simulink model "controller_autogen"  (R2022b)
settings: Solver=FixedStepDiscrete  StartTime=0.0  StopTime=inf  FixedStep=0.005  RelTol=1e-3
undefined symbols (not defined in the file): MI_STATUSES, simp_vd_interface, simp_vd_lib
libraries: battery_monitor_lib x1, driver_interface_lib x1, governor_lib x1, motor_interface_lib x1
settings Model: Creator=dr_pa  LastModifiedBy=LinF
settings OptimizationCC: DefaultParameterBehavior=Inlined  UseDivisionForNetSlopeComputation=on  GainParamInheritBuiltInType=on  UseFloatMulNetSlope=on  InlineInvariantSignals=on  PassReuseOutputArgsAs=Individual arguments  ZeroExternalMemoryAtStartup=off  ZeroInternalMemoryAtStartup=off  NoFixptDivByZeroProtection=on  EfficientFloat2IntCast=on  LifeSpan=1  OptimizeBlockOrder=speed  DifferentSizesBufferReuse=on  EfficientTunableParamExpr=on
settings DebuggingCC: ParameterTunabilityLossMsg=error
settings HardwareCC: ProdBitPerPointer=32  ProdBitPerSizeT=32  ProdBitPerPtrDiffT=32  ProdLargestAtomicInteger=Long  ProdLargestAtomicFloat=Double  ProdWordSize=32  ProdLongLongMode=on  ProdHWDeviceType=ARM Compatible->ARM Cortex-M
settings SFSimCC: MATLABDynamicMemAlloc=off
settings RTWCC: Description=Embedded Coder  SystemTargetFile=ert.tlc  GenCodeOnly=on  TemplateMakefile=ert_default_tmf
settings CodeAppCC: ForceParamTrailComments=on  IgnoreCustomStorageClasses=off  OperatorAnnotations=on  SimulinkDataObjDesc=on  SFDataObjDesc=on  CustomSymbolStrGlobalVar=rt$N$M  CustomSymbolStrType=$N$M  CustomSymbolStrFcn=$N$M$F  CustomSymbolStrMacro=$N$M  InsertBlockDesc=on
settings ERTTargetCC: TargetLangStandard=C99 (ISO)  IncludeMdlTerminateFcn=off  CombineSignalStateStructs=on  SupportAbsoluteTime=off  SupportComplex=off  SupportNonInlinedSFcns=on  InlinedParameterPlacement=NonHierarchical  ERTCustomFileTemplate=example_file_process.tlc  ERTFilePackagingFormat=CompactWithDataFile

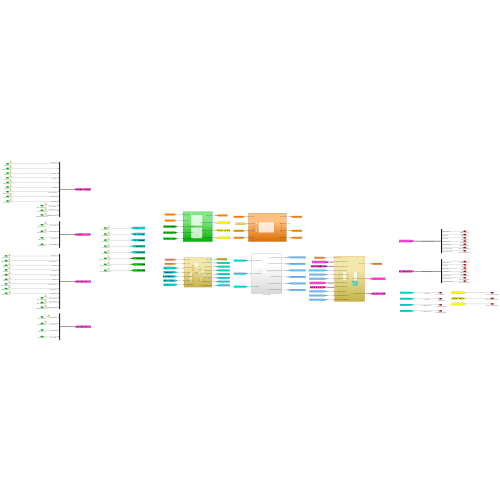
[thumbnail: Simulink's stored preview of the top-level diagram]
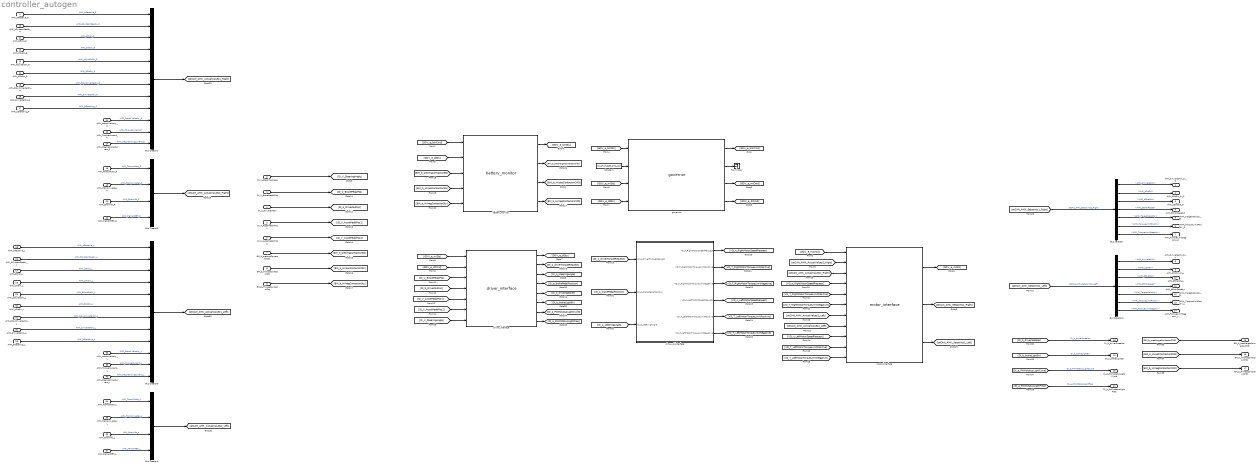
== system controller_autogen ==
  AMK_bReserve_R : Inport  OutDataTypeStr=boolean  Unit=uint64
  DI_V_SteeringAngle : Inport  Port=2  Unit=uint32
  DI_V_BrakePedalPos : Inport  Port=3  Unit=uint32
  DI_b_DriverButton : Inport  Port=4  Unit=uint32
  DI_V_AccelPedalPos1 : Inport  Port=5  Unit=uint32
  DI_V_AccelPedalPos2 : Inport  Port=6  Unit=uint32
  BM_b_prechrgContactorSts : Inport  Port=7  Unit=uint32
  BM_b_HVposContactorSts : Inport  Port=8  Unit=uint32
  BM_b_HVnegContactorSts : Inport  Port=9  Unit=uint32
  AMK_bSystemReady_R : Inport  Port=10  OutDataTypeStr=boolean  Unit=uint64
  AMK_bError_R : Inport  Port=11  OutDataTypeStr=boolean  Unit=uint64
  AMK_bWarn_R : Inport  Port=12  OutDataTypeStr=boolean  Unit=uint64
  AMK_bQuitDcOn_R : Inport  Port=13  OutDataTypeStr=boolean  Unit=uint64
  AMK_bDcOn_R : Inport  Port=14  OutDataTypeStr=boolean  Unit=uint64
  AMK_bQuitInverterOn_R : Inport  Port=15  OutDataTypeStr=boolean  Unit=uint64
  AMK_bInverterOn_R : Inport  Port=16  OutDataTypeStr=boolean  Unit=uint64
  AMK_bDerating_R : Inport  Port=17  OutDataTypeStr=boolean  Unit=uint64
  AMK_TempMotor_R : Inport  Port=18  OutDataTypeStr=int16  Unit=uint64
  AMK_TempInverter_R : Inport  Port=19  OutDataTypeStr=int16  Unit=uint64
  AMK_ErrorInfo_R : Inport  Port=20  OutDataTypeStr=uint16
  AMK_TempIGBT_R : Inport  Port=21  OutDataTypeStr=int16
  AMK_ActualVelocity_R : Inport  Port=22  OutDataTypeStr=int16  Unit=uint64
  AMK_TorqueCurrent_R : Inport  Port=23  OutDataTypeStr=int16  Unit=uint64
  AMK_MagnetizingCurrent_R : Inport  Port=24  OutDataTypeStr=int16  Unit=uint64
  AMK_bReserve_L : Inport  Port=25  OutDataTypeStr=boolean  Unit=uint64
  AMK_bSystemReady_L : Inport  Port=26  OutDataTypeStr=boolean  Unit=uint64
  AMK_bError_L : Inport  Port=27  OutDataTypeStr=boolean  Unit=uint64
  AMK_bWarn_L : Inport  Port=28  OutDataTypeStr=boolean  Unit=uint64
  AMK_bQuitDcOn_L : Inport  Port=29  OutDataTypeStr=boolean  Unit=uint64
  AMK_bDcOn_L : Inport  Port=30  OutDataTypeStr=boolean  Unit=uint64
  AMK_bQuitInverterOn_L : Inport  Port=31  OutDataTypeStr=boolean  Unit=uint64
  AMK_bInverterOn_L : Inport  Port=32  OutDataTypeStr=boolean  Unit=uint64
  AMK_bDerating_L : Inport  Port=33  OutDataTypeStr=boolean  Unit=uint64
  AMK_TempMotor_L : Inport  Port=34  OutDataTypeStr=int16  Unit=uint64
  AMK_TempInverter_L : Inport  Port=35  OutDataTypeStr=int16  Unit=uint64
  AMK_ErrorInfo_L : Inport  Port=36  OutDataTypeStr=uint16
  AMK_TempIGBT_L : Inport  Port=37  OutDataTypeStr=int16
  AMK_ActualVelocity_L : Inport  Port=38  OutDataTypeStr=int16  Unit=uint64
  AMK_TorqueCurrent_L : Inport  Port=39  OutDataTypeStr=int16  Unit=uint64
  AMK_MagnetizingCurrent_L : Inport  Port=40  OutDataTypeStr=int16  Unit=uint64
  Bus Creator1 : BusCreator  Inputs=12
  Bus Creator2 : BusCreator  Inputs=4
  Bus Creator3 : BusCreator  Inputs=12
  Bus Creator4 : BusCreator  Inputs=4
  Bus Selector : BusSelector  OutputSignals=AMK_bInverterOn,AMK_bDcOn,AMK_bEnable,AMK_bErrorReset,AMK_TargetVelocity,AMK_TorqueLimitPositiv,AMK_TorqueLimitNegativ
  Bus Selector1 : BusSelector  OutputSignals=AMK_bInverterOn,AMK_bDcOn,AMK_bEnable,AMK_bErrorReset,AMK_TargetVelocity,AMK_TorqueLimitPositiv,AMK_TorqueLimitNegativ
  Constant : Constant  Value=MI_STATUSES.STS_INIT  OutDataTypeStr=Enum: MI_STATUSES
  Terminator : Terminator
  battery_monitor : battery_monitor_lib/battery_monitor  SystemSampleTime=-1  VariantActivationTime=update diagram  Latency=0  AutoFrameSizeCalculation=off
  driver_interface : driver_interface_lib/driver_interface  SystemSampleTime=-1  VariantActivationTime=update diagram  Latency=0  AutoFrameSizeCalculation=off
  governor : governor_lib/governor  SystemSampleTime=-1  VariantActivationTime=update diagram  Latency=0  AutoFrameSizeCalculation=off
  motor_interface : motor_interface_lib/motor_interface  SystemSampleTime=-1  VariantActivationTime=update diagram  Latency=0  AutoFrameSizeCalculation=off
  simp_vd_interface : Subsystem  AncestorBlock=simp_vd_lib/simp_vd_interface
      settings: LibrarySourceBlock=simp_vd_lib/simp_vd_interface
  AMK_bInverterOn_tx_R : Outport
  AMK_bDcOn_tx_R : Outport  Port=2
  AMK_bEnable_R : Outport  Port=3
  AMK_bErrorReset_R : Outport  Port=4
  AMK_TargetVelocity_R : Outport  Port=5
  AMK_TorqueLimitPositiv_R : Outport  Port=6
  AMK_TorqueLimitNegativ_R : Outport  Port=7
  AMK_bInverterOn_tx_L : Outport  Port=8
  AMK_bDcOn_tx_L : Outport  Port=9
  AMK_bEnable_L : Outport  Port=10
  AMK_bErrorReset_L : Outport  Port=11
  AMK_TargetVelocity_L : Outport  Port=12
  AMK_TorqueLimitPositiv_L : Outport  Port=13
  AMK_TorqueLimitNegativ_L : Outport  Port=14
  BM_b_prechargeContactorCMD : Outport  Port=15
  BM_b_HVposContactorCMD : Outport  Port=16
  BM_b_HVnegContactorCMD : Outport  Port=17
  DI_b_driverSpeaker : Outport  Port=18
  DI_b_brakeLightEn : Outport  Port=19
  DI_p_PWMstatusLightCycle : Outport  Port=20
  DI_p_PWMstatusLightFreq : Outport  Port=21
  wires:
  driver_interface/3 -> [DI_p_steeringAngle]
  driver_interface/5 -> [DI_b_driverSpeaker]
  [GOV_e_miSts] -> governor/3
  [VD_T_RightMotorTorqueLimitPositive] -> motor_interface/5
  driver_interface/4 -> [DI_p_brakePedalPosition]
  BM_b_HVnegContactorSts/1 -> [BM_b_HVnegContactorSts]
  [ptCAN_AMK_Setpoints1_Left] -> Bus Selector1/1  "ptCAN_AMK_Setpoints1_Left"
  [DI_b_driverSpeaker] -> DI_b_driverSpeaker/1  "DI_b_driverSpeaker"
  [VD_T_RightMotorTorqueLimitNegative] -> motor_interface/6
  [GOV_e_bmCmd] -> battery_monitor/1
  driver_interface/2 -> [DI_p_driverTorqueRequest]
  DI_V_BrakePedalPos/1 -> [DI_V_BrakePedalPos]
  driver_interface/1 -> [GOV_e_diSts]
  Constant/1 -> governor/2
  [ptCAN_AMK_ActualValues2_Right] -> motor_interface/3
  [GOV_e_bmSts] -> governor/1
  battery_monitor/1 -> [GOV_e_bmSts]
  [VD_n_RightMotorSpeedRequest] -> motor_interface/4
  DI_V_AccelPedalPos2/1 -> [DI_V_AccelPedalPos2]
  governor/3 -> [GOV_e_miCmd]
  [GOV_e_diSts] -> governor/4
  [ptCAN_AMK_Setpoints1_Right] -> Bus Selector/1  "ptCAN_AMK_Setpoints1_Right"
  DI_b_DriverButton/1 -> [DI_b_DriverButton]
  BM_b_prechrgContactorSts/1 -> [BM_b_prechrgContactorSts]
  [GOV_e_miCmd] -> motor_interface/1
  governor/4 -> [GOV_e_diCmd]
  [ptCAN_AMK_ActualValues1_Right] -> motor_interface/2
  DI_V_AccelPedalPos1/1 -> [DI_V_AccelPedalPos1]
  governor/2 -> Terminator/1
  motor_interface/1 -> [GOV_e_miSts]
  BM_b_HVposContactorSts/1 -> [BM_b_HVposContactorSts]
  governor/1 -> [GOV_e_bmCmd]
  motor_interface/2 -> [ptCAN_AMK_Setpoints1_Right]
  DI_V_SteeringAngle/1 -> [DI_V_SteeringAngle]
  AMK_bSystemReady_R/1 -> Bus Creator1/2  "AMK_bSystemReady_R"
  AMK_bDerating_R/1 -> Bus Creator1/9  "AMK_bDerating_R"
  Bus Creator1/1 -> [ptCAN_AMK_ActualValues1_Right]
  AMK_bQuitDcOn_R/1 -> Bus Creator1/5  "AMK_bQuitDcOn_R"
  AMK_bQuitInverterOn_R/1 -> Bus Creator1/7  "AMK_bQuitInverterOn_R"
  AMK_TempInverter_R/1 -> Bus Creator2/2  "AMK_TempInverter_R"
  AMK_bDcOn_R/1 -> Bus Creator1/6  "AMK_bDcOn_R"
  AMK_bReserve_R/1 -> Bus Creator1/1  "AMK_bReserve_R"
  AMK_bWarn_R/1 -> Bus Creator1/4  "AMK_bWarn_R"
  AMK_ActualVelocity_R/1 -> Bus Creator1/10  "AMK_ActualVelocity_R"
  AMK_bError_R/1 -> Bus Creator1/3  "AMK_bError_R"
  AMK_TempMotor_R/1 -> Bus Creator2/1  "AMK_TempMotor_R"
  AMK_TorqueCurrent_R/1 -> Bus Creator1/11  "AMK_TorqueCurrent_R"
  AMK_TempIGBT_R/1 -> Bus Creator2/4  "AMK_TempIGBT_R"
  AMK_ErrorInfo_R/1 -> Bus Creator2/3  "AMK_ErrorInfo_R"
  AMK_MagnetizingCurrent_R/1 -> Bus Creator1/12  "AMK_MagnetizingCurrent_R"
  Bus Creator2/1 -> [ptCAN_AMK_ActualValues2_Right]
  AMK_bInverterOn_R/1 -> Bus Creator1/8  "AMK_bInverterOn_R"
  motor_interface/3 -> [ptCAN_AMK_Setpoints1_Left]
  [ptCAN_AMK_ActualValues1_Left] -> motor_interface/7
  [ptCAN_AMK_ActualValues2_Left] -> motor_interface/8
  [VD_n_LeftMotorSpeedRequest] -> motor_interface/9
  [VD_T_LeftMotorTorqueLimitPositive] -> motor_interface/10
  [VD_T_LeftMotorTorqueLimitNegative] -> motor_interface/11
  Bus Selector/4 -> AMK_bErrorReset_R/1  "<AMK_bErrorReset>"
  Bus Selector/5 -> AMK_TargetVelocity_R/1  "<AMK_TargetVelocity>"
  Bus Selector/1 -> AMK_bInverterOn_tx_R/1  "<AMK_bInverterOn>"
  Bus Selector/2 -> AMK_bDcOn_tx_R/1  "<AMK_bDcOn>"
  Bus Selector/6 -> AMK_TorqueLimitPositiv_R/1  "<AMK_TorqueLimitPositiv>"
  Bus Selector/3 -> AMK_bEnable_R/1  "<AMK_bEnable>"
  Bus Selector/7 -> AMK_TorqueLimitNegativ_R/1  "<AMK_TorqueLimitNegativ>"
  AMK_TorqueCurrent_L/1 -> Bus Creator3/11  "AMK_TorqueCurrent_L"
  AMK_ErrorInfo_L/1 -> Bus Creator4/3  "AMK_ErrorInfo_L"
  Bus Creator4/1 -> [ptCAN_AMK_ActualValues2_Left]
  AMK_bQuitInverterOn_L/1 -> Bus Creator3/7  "AMK_bQuitInverterOn_L"
  AMK_bSystemReady_L/1 -> Bus Creator3/2  "AMK_bSystemReady_L"
  AMK_MagnetizingCurrent_L/1 -> Bus Creator3/12  "AMK_MagnetizingCurrent_L"
  AMK_TempInverter_L/1 -> Bus Creator4/2  "AMK_TempInverter_L"
  AMK_bDerating_L/1 -> Bus Creator3/9  "AMK_bDerating_L"
  AMK_bQuitDcOn_L/1 -> Bus Creator3/5  "AMK_bQuitDcOn_L"
  AMK_TempIGBT_L/1 -> Bus Creator4/4  "AMK_TempIGBT_L"
  AMK_bDcOn_L/1 -> Bus Creator3/6  "AMK_bDcOn_L"
  AMK_TempMotor_L/1 -> Bus Creator4/1  "AMK_TempMotor_L"
  Bus Creator3/1 -> [ptCAN_AMK_ActualValues1_Left]
  AMK_bError_L/1 -> Bus Creator3/3  "AMK_bError_L"
  AMK_bWarn_L/1 -> Bus Creator3/4  "AMK_bWarn_L"
  AMK_ActualVelocity_L/1 -> Bus Creator3/10  "AMK_ActualVelocity_L"
  AMK_bReserve_L/1 -> Bus Creator3/1  "AMK_bReserve_L"
  AMK_bInverterOn_L/1 -> Bus Creator3/8  "AMK_bInverterOn_L"
  Bus Selector1/4 -> AMK_bErrorReset_L/1  "<AMK_bErrorReset>"
  Bus Selector1/1 -> AMK_bInverterOn_tx_L/1  "<AMK_bInverterOn>"
  Bus Selector1/3 -> AMK_bEnable_L/1  "<AMK_bEnable>"
  Bus Selector1/7 -> AMK_TorqueLimitNegativ_L/1  "<AMK_TorqueLimitNegativ>"
  Bus Selector1/6 -> AMK_TorqueLimitPositiv_L/1  "<AMK_TorqueLimitPositiv>"
  Bus Selector1/5 -> AMK_TargetVelocity_L/1  "<AMK_TargetVelocity>"
  Bus Selector1/2 -> AMK_bDcOn_tx_L/1  "<AMK_bDcOn>"
  [DI_p_brakePedalPosition] -> simp_vd_interface/2(DI_p_brakePedalPosition)
  simp_vd_interface/4(VD_n_LeftMotorSpeedRequest) -> [VD_n_LeftMotorSpeedRequest]
  simp_vd_interface/5(VD_T_LeftMotorTorqueLimitPositive) -> [VD_T_LeftMotorTorqueLimitPositive]
  simp_vd_interface/1(VD_n_RightMotorSpeedRequest) -> [VD_n_RightMotorSpeedRequest]
  [DI_p_steeringAngle] -> simp_vd_interface/3(DI_p_steeringAngle)
  simp_vd_interface/6(VD_T_LeftMotorTorqueLimitNegative) -> [VD_T_LeftMotorTorqueLimitNegative]
  [DI_p_driverTorqueRequest] -> simp_vd_interface/1(DI_p_driverTorqueRequest)
  simp_vd_interface/3(VD_T_RightMotorTorqueLimitNegative) -> [VD_T_RightMotorTorqueLimitNegative]
  simp_vd_interface/2(VD_T_RightMotorTorqueLimitPositive) -> [VD_T_RightMotorTorqueLimitPositive]
  [BM_b_prechrgContactorSts] -> battery_monitor/3
  [BM_b_HVposContactorSts] -> battery_monitor/4
  [BM_b_HVnegContactorSts] -> battery_monitor/5
  [GOV_e_diSts] -> battery_monitor/2
  battery_monitor/2 -> [BM_b_prechargeContactorCMD]
  battery_monitor/3 -> [BM_b_HVposContactorCMD]
  battery_monitor/4 -> [BM_b_HVnegContactorCMD]
  driver_interface/6 -> [DI_b_brakeLightEn]
  driver_interface/7 -> [DI_p_PWMstatusLightCycle]
  driver_interface/8 -> [DI_p_PWMstatusLightFreq]
  [BM_b_prechargeContactorCMD] -> BM_b_prechargeContactorCMD/1
  [BM_b_HVposContactorCMD] -> BM_b_HVposContactorCMD/1
  [BM_b_HVnegContactorCMD] -> BM_b_HVnegContactorCMD/1
  [DI_b_brakeLightEn] -> DI_b_brakeLightEn/1  "DI_b_brakeLightEn"
  [DI_p_PWMstatusLightCycle] -> DI_p_PWMstatusLightCycle/1  "DI_p_PWMstatusLightCycle"
  [DI_p_PWMstatusLightFreq] -> DI_p_PWMstatusLightFreq/1  "DI_p_PWMstatusLightFreq"
  [GOV_e_diCmd] -> driver_interface/2
  [DI_V_BrakePedalPos] -> driver_interface/3
  [DI_b_DriverButton] -> driver_interface/4
  [DI_V_AccelPedalPos1] -> driver_interface/5
  [DI_V_AccelPedalPos2] -> driver_interface/6
  [DI_V_SteeringAngle] -> driver_interface/7
  [GOV_e_miSts] -> driver_interface/1

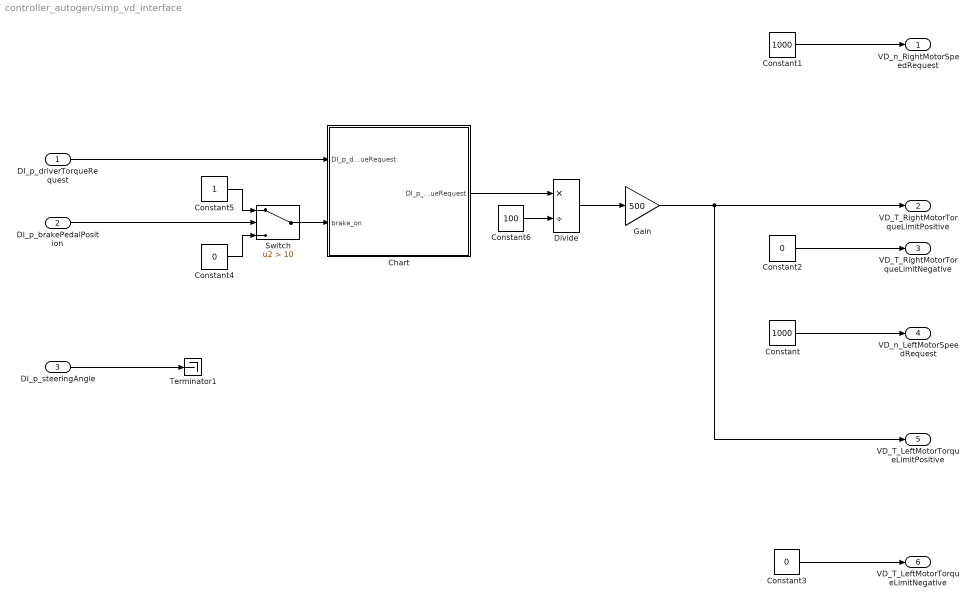
== system controller_autogen/simp_vd_interface ==
  DI_p_driverTorqueRequest : Inport
  DI_p_brakePedalPosition : Inport  Port=2
  DI_p_steeringAngle : Inport  Port=3
  Chart : Stateflow chart  TreatAsAtomicUnit=on
  Constant : Constant  Value=1000
  Constant1 : Constant  Value=1000
  Constant2 : Constant  Value=0
  Constant3 : Constant  Value=0
  Constant4 : Constant  Value=0
  Constant5 : Constant
  Constant6 : Constant  Value=100
  Divide : Product  Inputs=*/
  Gain : Gain  Gain=500
  Switch : Switch  Criteria=u2 > Threshold  Threshold=10  SaturateOnIntegerOverflow=off  InputSameDT=off
  Terminator1 : Terminator
  VD_n_RightMotorSpeedRequest : Outport
  VD_T_RightMotorTorqueLimitPositive : Outport  Port=2
  VD_T_RightMotorTorqueLimitNegative : Outport  Port=3
  VD_n_LeftMotorSpeedRequest : Outport  Port=4
  VD_T_LeftMotorTorqueLimitPositive : Outport  Port=5
  VD_T_LeftMotorTorqueLimitNegative : Outport  Port=6
  wires:
  DI_p_steeringAngle/1 -> Terminator1/1
  Constant/1 -> VD_n_LeftMotorSpeedRequest/1
  Constant1/1 -> VD_n_RightMotorSpeedRequest/1
  Constant2/1 -> VD_T_RightMotorTorqueLimitNegative/1
  Constant3/1 -> VD_T_LeftMotorTorqueLimitNegative/1
  Constant4/1 -> Switch/3
  Constant5/1 -> Switch/1
  Switch/1 -> Chart/2(brake_on)
  DI_p_brakePedalPosition/1 -> Switch/2
  DI_p_driverTorqueRequest/1 -> Chart/1(DI_p_driverTorqueRequest)
  Constant6/1 -> Divide/2
  Chart/1(DI_p_motorTorqueRequest) -> Divide/1
  Divide/1 -> Gain/1
  Gain/1 -> VD_T_LeftMotorTorqueLimitPositive/1, VD_T_RightMotorTorqueLimitPositive/1

== stateflow chart controller_autogen/simp_vd_interface/Chart ==
  state Run
    en, du:
    DI_p_motorTorqueRequest = DI_p_driverTorqueRequest;
  state Stop
    en, du:
    DI_p_motorTorqueRequest = 0;
  (default) -> Run
  Run -> Stop : [DI_p_driverTorqueRequest >= 20 && brake_on]
  Stop -> Run : [DI_p_driverTorqueRequest < 5 && ~brake_on]
  data: DI_p_driverTorqueRequest input; brake_on input; DI_p_motorTorqueRequest output
